simulink model "MBD_Switch_Case_Action_Subsystem"  (R2021b)
settings: Solver=FixedStepDiscrete  StartTime=0.0  StopTime=10.0  FixedStep=0.001  RelTol=1e-3
libraries: simulink x1
settings Model: NumberOfSteps=100  Creator=waleed.elshemy  LastModifiedBy=waleed.elshemy
settings OptimizationCC: DefaultParameterBehavior=Inlined  UseDivisionForNetSlopeComputation=on  GainParamInheritBuiltInType=on  UseFloatMulNetSlope=on  InlineInvariantSignals=on  PassReuseOutputArgsAs=Individual arguments  ZeroExternalMemoryAtStartup=off  ZeroInternalMemoryAtStartup=off  NoFixptDivByZeroProtection=on  EfficientFloat2IntCast=on  LifeSpan=1  OptimizeBlockOrder=speed  DifferentSizesBufferReuse=on  EfficientTunableParamExpr=on
settings DebuggingCC: ParameterTunabilityLossMsg=error
settings HardwareCC: ProdLongLongMode=on
settings SFSimCC: MATLABDynamicMemAlloc=off
settings RTWCC: Description=Embedded Coder  SystemTargetFile=ert.tlc  TemplateMakefile=ert_default_tmf
settings CodeAppCC: ForceParamTrailComments=on  IgnoreCustomStorageClasses=off  OperatorAnnotations=on  SimulinkDataObjDesc=on  SFDataObjDesc=on  CustomSymbolStrGlobalVar=rt$N$M  CustomSymbolStrType=$N$M  CustomSymbolStrFcn=$N$M$F  CustomSymbolStrMacro=$N$M  InsertBlockDesc=on
settings ERTTargetCC: TargetLangStandard=C99 (ISO)  GenerateSampleERTMain=on  IncludeMdlTerminateFcn=off  CombineSignalStateStructs=on  SupportComplex=off  SupportContinuousTime=on  InlinedParameterPlacement=NonHierarchical  ERTCustomFileTemplate=example_file_process.tlc  ERTFilePackagingFormat=CompactWithDataFile

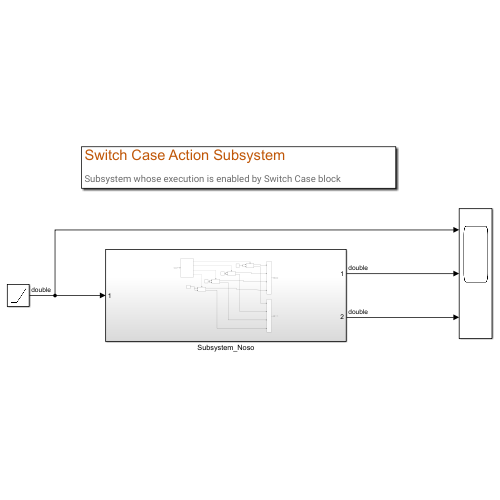
[thumbnail: Simulink's stored preview of the top-level diagram]
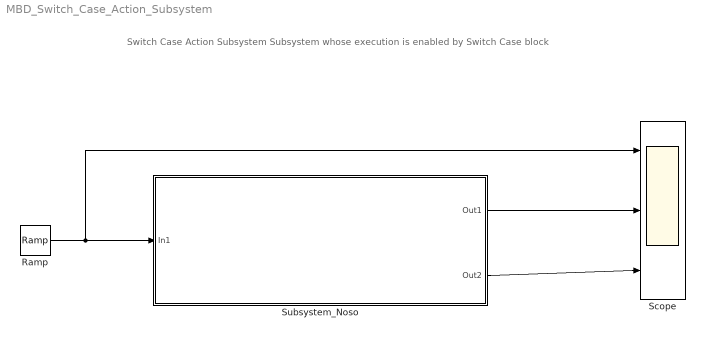
== system MBD_Switch_Case_Action_Subsystem ==
  note: Switch Case Action Subsystem
      | Subsystem whose execution is enabled by Switch Case block
  Ramp : simulink/Sources/Ramp  slope=1  start=0  InitialOutput=0
  Scope : Scope  NumInputPorts=3
  Subsystem_Noso : Subsystem
  wires:
  Ramp/1 -> Scope/1, Subsystem_Noso/1(In1)
  Subsystem_Noso/1(Out1) -> Scope/2
  Subsystem_Noso/2(Out2) -> Scope/3

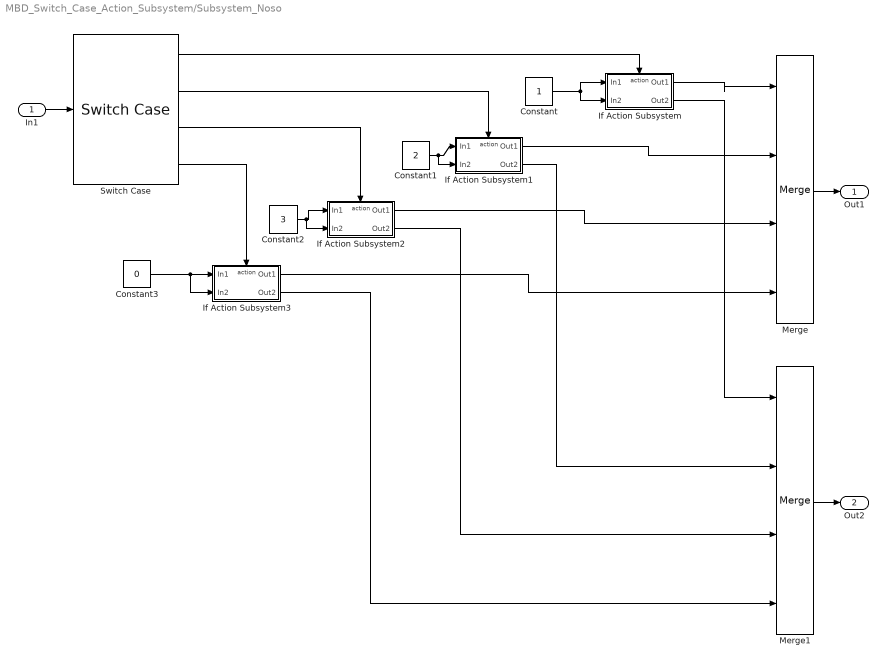
== system MBD_Switch_Case_Action_Subsystem/Subsystem_Noso ==
  In1 : Inport
  Constant : Constant
  Constant1 : Constant  Value=2
  Constant2 : Constant  Value=3
  Constant3 : Constant  Value=0
  If Action Subsystem : Subsystem  TreatAsAtomicUnit=on
  If Action Subsystem1 : Subsystem  TreatAsAtomicUnit=on
  If Action Subsystem2 : Subsystem  TreatAsAtomicUnit=on
  If Action Subsystem3 : Subsystem  TreatAsAtomicUnit=on
  Merge : Merge  Inputs=4
  Merge1 : Merge  Inputs=4
  Switch Case : SwitchCase  CaseConditions={1,3,5}
  Out1 : Outport
  Out2 : Outport  Port=2
  wires:
  Switch Case/4 -> If Action Subsystem3/Action
  Constant/1 -> If Action Subsystem/1(In1), If Action Subsystem/2(In2)
  Constant2/1 -> If Action Subsystem2/2(In2), If Action Subsystem2/1(In1)
  Constant3/1 -> If Action Subsystem3/2(In2), If Action Subsystem3/1(In1)
  If Action Subsystem3/1(Out1) -> Merge/4
  If Action Subsystem2/1(Out1) -> Merge/3
  Switch Case/1 -> If Action Subsystem/Action
  Switch Case/2 -> If Action Subsystem1/Action
  Constant1/1 -> If Action Subsystem1/2(In2), If Action Subsystem1/1(In1)
  If Action Subsystem1/1(Out1) -> Merge/2
  Merge/1 -> Out1/1
  If Action Subsystem/1(Out1) -> Merge/1
  Switch Case/3 -> If Action Subsystem2/Action
  In1/1 -> Switch Case/1
  If Action Subsystem/2(Out2) -> Merge1/1
  If Action Subsystem1/2(Out2) -> Merge1/2
  If Action Subsystem2/2(Out2) -> Merge1/3
  If Action Subsystem3/2(Out2) -> Merge1/4
  Merge1/1 -> Out2/1

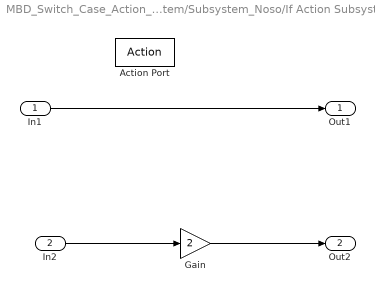
== system MBD_Switch_Case_Action_Subsystem/Subsystem_Noso/If Action Subsystem ==
  In1 : Inport
  In2 : Inport  Port=2
  Action Port : ActionPort  InitializeStates=reset  ActionPortLabel=case [ 1 ]:
  Gain : Gain  Gain=2
  Out1 : Outport
  Out2 : Outport  Port=2
  wires:
  In1/1 -> Out1/1
  Gain/1 -> Out2/1
  In2/1 -> Gain/1

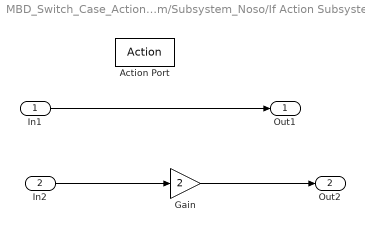
== system MBD_Switch_Case_Action_Subsystem/Subsystem_Noso/If Action Subsystem1 ==
  In1 : Inport
  In2 : Inport  Port=2
  Action Port : ActionPort  ActionPortLabel=case [ 3 ]:
  Gain : Gain  Gain=2
  Out1 : Outport
  Out2 : Outport  Port=2
  wires:
  In1/1 -> Out1/1
  Gain/1 -> Out2/1
  In2/1 -> Gain/1

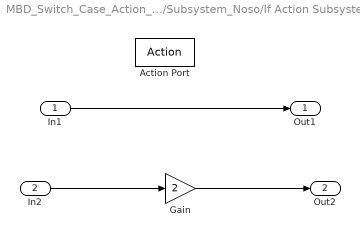
== system MBD_Switch_Case_Action_Subsystem/Subsystem_Noso/If Action Subsystem2 ==
  In1 : Inport
  In2 : Inport  Port=2
  Action Port : ActionPort  ActionPortLabel=case [ 5 ]:
  Gain : Gain  Gain=2
  Out1 : Outport
  Out2 : Outport  Port=2
  wires:
  In1/1 -> Out1/1
  Gain/1 -> Out2/1
  In2/1 -> Gain/1

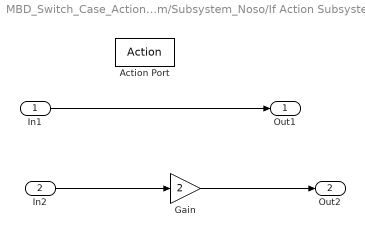
== system MBD_Switch_Case_Action_Subsystem/Subsystem_Noso/If Action Subsystem3 ==
  In1 : Inport
  In2 : Inport  Port=2
  Action Port : ActionPort  ActionPortLabel=default:
  Gain : Gain  Gain=2
  Out1 : Outport
  Out2 : Outport  Port=2
  wires:
  In1/1 -> Out1/1
  Gain/1 -> Out2/1
  In2/1 -> Gain/1
